simulink model "cl_fforward"  (R2024b)
settings: Solver=ode23t  StartTime=0.0  StopTime=5  RelTol=1e-3  EnableMultiTasking=on
values from neighbouring files (symbols this model uses):
  Kd = 5    [controlled_robot_def_ctorque.m]    (also in controlled_robot_def_freedfwrd.m = [5])
  Kp = [50 50 50]    [controlled_robot_def_Nested.m]    (also in controlled_robot_def_ctorque.m = 20; controlled_robot_def_freedfwrd.m = [100])
  q_inicial = [0 0 0]    [circle_drawing.m]    (also in controlled_robot_def_Nested.m; controlled_robot_def_PD.m; controlled_robot_def_PID.m; controlled_robot_def_ctorque.m)
  qf = [pi/2 pi/2 pi/2]    [controlled_robot_def_Nested.m]    (also in controlled_robot_def_PD.m = [pi/2 pi/4 pi/4]; controlled_robot_def_PID.m; controlled_robot_def_ctorque.m; controlled_robot_def_freedfwrd.m)
  robot_3dof = SerialLink(L, 'name', 'Robot 3-DOF')    [circle_drawing.m]    (also in controlled_robot_def_Nested.m; controlled_robot_def_PD.m; controlled_robot_def_PID.m; controlled_robot_def_ctorque.m)
  unc = 0.2    [controlled_robot_def_Nested.m]    (also in controlled_robot_def_PD.m; controlled_robot_def_PID.m; controlled_robot_def_ctorque.m = 0; controlled_robot_def_freedfwrd.m)
libraries: roblocks x3
settings Model: Creator=corkep  LastModifiedBy=pablo
settings SolverCC: AlgebraicLoopSolver=TrustRegion
settings DataIOCC: LimitDataPoints=on  SaveFormat=Array  SignalLoggingSaveFormat=ModelDataLogs  TimeSaveName=t  OutputSaveName=y  ReturnWorkspaceOutputsName=fforward
settings OptimizationCC: ExpressionDepthLimit=2147483647  LifeSpan=inf
settings DebuggingCC: UnderspecifiedInitializationDetection=Classic  MergeDetectMultiDrivingBlocksExec=none  SolverPrmCheckMsg=warning  FcnCallInpInsideContextMsg=warning  UnconnectedInputMsg=warning  UnconnectedOutputMsg=warning  UnconnectedLineMsg=warning  AllowSymbolicDim=off  StateNameClashWarn=warning  SFUnexpectedBacktrackingDiag=warning  SFNoUnconditionalDefaultTransitionDiag=warning  SFExecutionAtInitializationDiag=none  ArithmeticOperatorsInVariantConditions=warning
settings HardwareCC: ProdBitPerPointer=32  ProdBitPerSizeT=32  ProdBitPerPtrDiffT=32  ProdLargestAtomicFloat=None  ProdIntDivRoundTo=Undefined  ProdEndianess=Unspecified  ProdWordSize=32  ProdHWDeviceType=32-bit Generic
settings ModelReferenceCC: EnableRefExpFcnMdlSchedulingChecks=on  PropagateSignalLabelsOutOfModel=off
settings SFSimCC: SimUseLocalCustomCode=off  CustomCodeUndefinedFunction=UseInterfaceOnly
settings RTWCC: RTWUseLocalCustomCode=off  GPUComputeCapability=3.5
settings CodeAppCC: StateflowObjectComments=on
settings GRTTargetCC: TargetLangStandard=C89/C90 (ANSI)  CombineOutputUpdateFcns=off  GRTInterface=on
settings ConfigComp: CovMetricSettings=dw  CovSaveCumulativeToWorkspaceVar=on  CovSaveSingleToWorkspaceVar=on  CovExternalEMLEnable=off

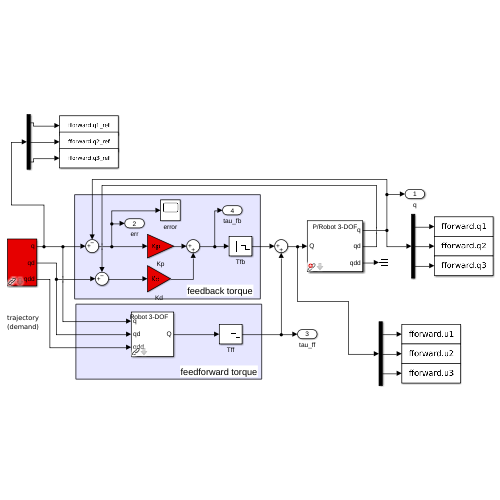
[thumbnail: Simulink's stored preview of the top-level diagram]
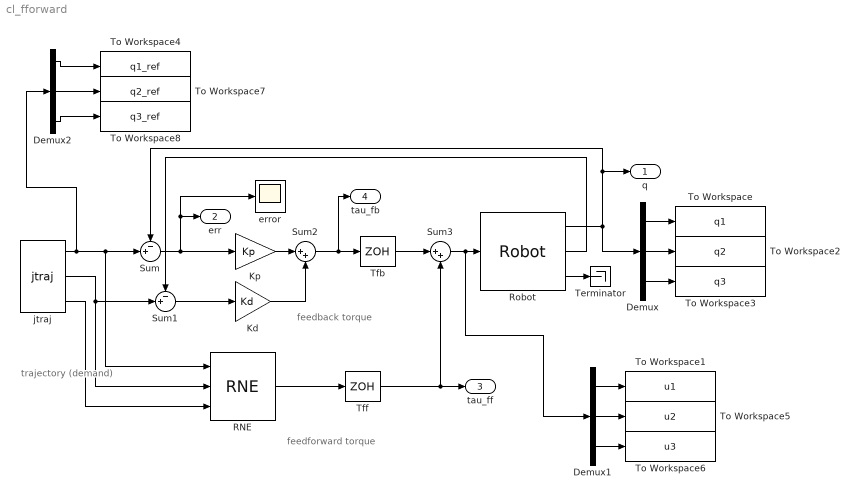
== system cl_fforward ==
  note: feedforward torque
  note: trajectory
      | (demand)
  note: feedback torque
  Demux : Demux  Outputs=3
  Demux1 : Demux  Outputs=3
  Demux2 : Demux  Outputs=3
  Kd : Gain  Gain=Kd  SaturateOnIntegerOverflow=on  OutDataTypeStr=Inherit: Same as input  ParamDataTypeStr=Inherit: Same as input
  Kp : Gain  Gain=Kp  SaturateOnIntegerOverflow=on  OutDataTypeStr=Inherit: Same as input  ParamDataTypeStr=Inherit: Same as input
  RNE : roblocks/Arm/RNE  robot=robot_3dof  grav=[0 0 9.81]
  Robot : roblocks/Arm/Robot  robot=robot_3dof.perturb(unc)  q0=q_inicial
      link override Integrator1: InitialCondition=q0
  Sum : Sum  Inputs=-+|  InputSameDT=on  SaturateOnIntegerOverflow=on  OutDataTypeStr=Inherit: Same as first input
  Sum1 : Sum  Inputs=-+|  InputSameDT=on  SaturateOnIntegerOverflow=on  OutDataTypeStr=Inherit: Same as first input
  Sum2 : Sum  Inputs=|++  InputSameDT=on  SaturateOnIntegerOverflow=on  OutDataTypeStr=Inherit: Same as first input
  Sum3 : Sum  Inputs=|++  InputSameDT=on  SaturateOnIntegerOverflow=on  OutDataTypeStr=Inherit: Same as first input
  Terminator : Terminator
  Tfb : ZeroOrderHold  SampleTime=0.002
  Tff : ZeroOrderHold  SampleTime=0.05
  To Workspace : ToWorkspace  VariableName=q1  SaveFormat=Timeseries  SampleTime=-1
  To Workspace1 : ToWorkspace  VariableName=u1  SaveFormat=Timeseries  SampleTime=-1
  To Workspace2 : ToWorkspace  VariableName=q2  SaveFormat=Timeseries  SampleTime=-1
  To Workspace3 : ToWorkspace  VariableName=q3  SaveFormat=Timeseries  SampleTime=-1
  To Workspace4 : ToWorkspace  VariableName=q1_ref  SaveFormat=Timeseries  SampleTime=-1
  To Workspace5 : ToWorkspace  VariableName=u2  SaveFormat=Timeseries  SampleTime=-1
  To Workspace6 : ToWorkspace  VariableName=u3  SaveFormat=Timeseries  SampleTime=-1
  To Workspace7 : ToWorkspace  VariableName=q2_ref  SaveFormat=Timeseries  SampleTime=-1
  To Workspace8 : ToWorkspace  VariableName=q3_ref  SaveFormat=Timeseries  SampleTime=-1
  error : Scope
  jtraj : roblocks/Toolbox/jtraj  q0=[q_inicial(1) q_inicial(2) q_inicial(3)]  qf=[qf(1) qf(2) qf(3)]  tmax=Tmax  ts=0.002
  q : Outport
  err : Outport  Port=2
  tau_ff : Outport  Port=3
  tau_fb : Outport  Port=4
  wires:
  Demux1/1 -> To Workspace1/1
  Sum/1 -> error/1, err/1, Kp/1
  Tfb/1 -> Sum3/1
  Robot/3 -> Terminator/1
  Demux1/3 -> To Workspace6/1
  Demux/1 -> To Workspace/1
  Robot/2 -> Sum1/1
  Demux2/2 -> To Workspace7/1
  Sum1/1 -> Kd/1
  RNE/1 -> Tff/1
  Demux1/2 -> To Workspace5/1
  Demux/3 -> To Workspace3/1
  jtraj/3 -> RNE/3
  Demux/2 -> To Workspace2/1
  Tff/1 -> Sum3/2, tau_ff/1
  Demux2/3 -> To Workspace8/1
  jtraj/2 -> Sum1/2, RNE/2
  Sum2/1 -> Tfb/1, tau_fb/1
  Robot/1 -> Demux/1, Sum/1, q/1
  Kd/1 -> Sum2/2
  Demux2/1 -> To Workspace4/1
  Kp/1 -> Sum2/1
  jtraj/1 -> Demux2/1, RNE/1, Sum/2
  Sum3/1 -> Demux1/1, Robot/1
